simulink model "LCK_DanishV01"  (R2018b)
settings: Solver=FixedStepDiscrete  StartTime=0.0  StopTime=inf  FixedStep=0.01  RelTol=1e-3
PostLoadFcn:
  | if any(exist('dsrtsu_mdlpostloadfcn', 'file') ~= 0), dsrtsu_mdlpostloadfcn('Execute', bdroot); end
values from neighbouring files (symbols this model uses):
  C_DEG2RAD = 0.0175    [LCK_Macro.sldd]
  C_KPH2MPS = 0.2778    [LCK_Macro.sldd]
  C_NEARZERO = 0.0001    [LCK_Macro.sldd]
  C_ONE = 1.0    [LCK_Macro.sldd]
  C_RAD2DEG = 57.2958    [LCK_Macro.sldd]
  C_ZERO = 0.0    [LCK_Macro.sldd]
  k_accel_pedal_pos_per_speed_x : value not decoded    [LCK_LogicPara.sldd]
  k_accel_pedal_pos_per_speed_z : value not decoded    [LCK_LogicPara.sldd]
  k_brake_suprress_hold = 1000.0    [LCK_LogicPara.sldd]
  k_driver_appl_torque_filt = 50.0    [LCK_LogicPara.sldd]
  k_driver_suppression_hold_time = 3000.0    [LCK_LogicPara.sldd]
  k_hands_on_wheel_hold_msec = 500.0    [LCK_LogicPara.sldd]
  k_hands_on_wheel_torque_hi = 0.2    [LCK_LogicPara.sldd]
  k_hands_on_wheel_torque_lo = 0.15    [LCK_LogicPara.sldd]
  k_handsoff_delay_cycles = 50.0    [LCK_LogicPara.sldd]
  k_handsoff_torq_Lo_CR = 0.3    [LCK_LogicPara.sldd]
  k_handson_delay_cycles = 5.0    [LCK_LogicPara.sldd]
  k_HighAccel_suppress_hold = 3000.0    [LCK_LogicPara.sldd]
  k_HLR_suprress_hold = 3000.0    [LCK_LogicPara.sldd]
  k_hs_StrAng_CR_threshold_z : value not decoded    [LCK_LogicPara.sldd]
  k_LC_Exit_Switch = 0.0    [LCK_LogicPara.sldd]
  k_LCG_Configured = 1.0    [LCK_LogicPara.sldd]
  k_LCK_A0_Rdy2Act_UseConst = 0.0    [LCK_LogicPara.sldd]
  k_LCK_A0Fac_ActSta : value not decoded    [LCK_CtrlPara.sldd]
  k_LCK_A0Fac_DrvStm : value not decoded    [LCK_CtrlPara.sldd]
  k_LCK_A0Shift_LftCurv : value not decoded    [LCK_CtrlPara.sldd]
  k_LCK_A0Shift_RgtCurv : value not decoded    [LCK_CtrlPara.sldd]
  k_LCK_A0Shift_StraLan = 0.0    [LCK_CtrlPara.sldd]
  k_LCK_A0ShiftFac_Dy_LftCurv : value not decoded    [LCK_CtrlPara.sldd]
  k_LCK_A0ShiftFac_Dy_RgtCurv : value not decoded    [LCK_CtrlPara.sldd]
  k_LCK_A0ShiftFac_Vspd : value not decoded    [LCK_CtrlPara.sldd]
  k_LCK_accel_inhibit_thold = 35.0    [LCK_LogicPara.sldd]
  k_LCK_Active2Ready_Mask = 255.0    [LCK_LogicPara.sldd]
  k_LCK_CvatRateBks : value not decoded    [LCK_CtrlPara.sldd]
  k_LCK_CvatrBks : value not decoded    [LCK_CtrlPara.sldd]
  k_LCK_DFac_Dy : value not decoded    [LCK_CtrlPara.sldd]
  k_LCK_DFac_Dy_Curv : value not decoded    [LCK_CtrlPara.sldd]
  k_LCK_DFac_HaCurCen : value not decoded    [LCK_CtrlPara.sldd]
  k_LCK_DFac_HaCurSid : value not decoded    [LCK_CtrlPara.sldd]
  k_LCK_DFac_HadCurCen : value not decoded    [LCK_CtrlPara.sldd]
  k_LCK_DFac_HadCurSid : value not decoded    [LCK_CtrlPara.sldd]
  k_LCK_DFac_HadStrCen : value not decoded    [LCK_CtrlPara.sldd]
  k_LCK_DFac_HadStrSid : value not decoded    [LCK_CtrlPara.sldd]
  k_LCK_DFac_HaStrCen : value not decoded    [LCK_CtrlPara.sldd]
  k_LCK_DFac_HaStrSid : value not decoded    [LCK_CtrlPara.sldd]
  k_LCK_DFac_Rad : value not decoded    [LCK_CtrlPara.sldd]
  k_LCK_DFac_SA_CurCen : value not decoded    [LCK_CtrlPara.sldd]
  k_LCK_DFac_SA_CurSid : value not decoded    [LCK_CtrlPara.sldd]
  k_LCK_DFac_SA_StrCen : value not decoded    [LCK_CtrlPara.sldd]
  k_LCK_DFac_SA_StrSid : value not decoded    [LCK_CtrlPara.sldd]
  k_LCK_DFac_SS_CurCen : value not decoded    [LCK_CtrlPara.sldd]
  k_LCK_DFac_SS_CurSid : value not decoded    [LCK_CtrlPara.sldd]
  k_LCK_DFac_SS_StrCen : value not decoded    [LCK_CtrlPara.sldd]
  k_LCK_DFac_SS_StrSid : value not decoded    [LCK_CtrlPara.sldd]
  k_LCK_DFac_Vspd : value not decoded    [LCK_CtrlPara.sldd]
  k_LCK_DlyTm_DrvStim = 0.2    [LCK_CtrlPara.sldd]
  k_LCK_DTermMax = 2.0    [LCK_CtrlPara.sldd]
  k_LCK_DyBks_Curv : value not decoded    [LCK_CtrlPara.sldd]
  k_LCK_Enable_POOnly = 1.0    [LCK_LogicPara.sldd]
  k_LCK_Entry_DistBuffer = 0.1    [LCK_LogicPara.sldd]
  k_LCK_Fac_Vspd2RngThr_FalRec = 0.23    [LCK_CtrlPara.sldd]
  k_LCK_Ffw_CvatSwh = 0.0    [LCK_CtrlPara.sldd]
  k_LCK_Ffw_DyBks : value not decoded    [LCK_CtrlPara.sldd]
  k_LCK_Ffw_TimCon_CmdFlt = 0.0    [LCK_CtrlPara.sldd]
  k_LCK_FfwDeltaFac_Rad_Lft : value not decoded    [LCK_CtrlPara.sldd]
  k_LCK_FfwDeltaFac_Rad_Rgt : value not decoded    [LCK_CtrlPara.sldd]
  k_LCK_FfwDeltaFac_Vspd : value not decoded    [LCK_CtrlPara.sldd]
  k_LCK_FfwFac_CvatRate_Lft : value not decoded    [LCK_CtrlPara.sldd]
  k_LCK_FfwFac_CvatRate_Rgt : value not decoded    [LCK_CtrlPara.sldd]
  k_LCK_FfwFac_Dy : value not decoded    [LCK_CtrlPara.sldd]
  k_LCK_FfwFac_Rad_Lft : value not decoded    [LCK_CtrlPara.sldd]
  k_LCK_FfwFac_Rad_Rgt : value not decoded    [LCK_CtrlPara.sldd]
  k_LCK_FfwFac_Vspd : value not decoded    [LCK_CtrlPara.sldd]
  k_LCK_FfwTorq_Cvat : value not decoded    [LCK_CtrlPara.sldd]
  k_LCK_HAFac_ActSta : value not decoded    [LCK_CtrlPara.sldd]
  k_LCK_HAFac_DrvStm : value not decoded    [LCK_CtrlPara.sldd]
  k_LCK_HaloTime = 2000.0    [LCK_LogicPara.sldd]
  k_LCK_HaloTime_Switch = 0.0    [LCK_LogicPara.sldd]
  k_LCK_HARFac_ActSta : value not decoded    [LCK_CtrlPara.sldd]
  k_LCK_HARFac_DrvStm : value not decoded    [LCK_CtrlPara.sldd]
  k_LCK_Hed_DyBks : value not decoded    [LCK_CtrlPara.sldd]
  k_LCK_HedAngDiffX : value not decoded    [LCK_CtrlPara.sldd]
  k_LCK_HedAngRateDiffX : value not decoded    [LCK_CtrlPara.sldd]
  k_LCK_HndsOnWhel_DlyTm_Idl2Rdy = 0.0    [LCK_LogicPara.sldd]
  k_LCK_host_veh_width = 1.86    [LCK_LogicPara.sldd]
  k_LCK_Idle2Ready_Mask = 239.0    [LCK_LogicPara.sldd]
  k_LCK_Junc_SusTime = 1.0    [LCK_LogicPara.sldd]
  k_LCK_KpKdDecSlopeLmt = 10.0    [LCK_CtrlPara.sldd]
  k_LCK_KpKdIncSlopeLmt = 5.0    [LCK_CtrlPara.sldd]
  k_LCK_Lat_Ctrl_DFac_Lft = 1.0    [LCK_CtrlPara.sldd]
  k_LCK_Lat_Ctrl_DFac_Rgt = 1.05    [LCK_CtrlPara.sldd]
  k_LCK_Lat_Ctrl_Kd = 0.8    [LCK_CtrlPara.sldd]
  k_LCK_Lat_Ctrl_Ki = 0.5    [LCK_CtrlPara.sldd]
  k_LCK_Lat_Ctrl_Kp = 0.7    [LCK_CtrlPara.sldd]
  k_LCK_Lat_Ctrl_Kp_NearGain = 0.7    [LCK_CtrlPara.sldd]
  k_LCK_Lat_Ctrl_PFac_Lft = 1.0    [LCK_CtrlPara.sldd]
  k_LCK_Lat_Ctrl_PFac_Rgt = 1.05    [LCK_CtrlPara.sldd]
  k_LCK_Lat_Ctrl_TimCon_CmdFlt = 5.0    [LCK_CtrlPara.sldd]
  k_LCK_Lat_DFac_Rad : value not decoded    [LCK_CtrlPara.sldd]
  k_LCK_Lat_DFac_SS_Cur : value not decoded    [LCK_CtrlPara.sldd]
  k_LCK_Lat_DFac_SS_Str : value not decoded    [LCK_CtrlPara.sldd]
  k_LCK_Lat_DFac_Vspd : value not decoded    [LCK_CtrlPara.sldd]
  k_LCK_Lat_DyBks : value not decoded    [LCK_CtrlPara.sldd]
  k_LCK_Lat_IFac_Rad : value not decoded    [LCK_CtrlPara.sldd]
  k_LCK_Lat_IFac_Vspd : value not decoded    [LCK_CtrlPara.sldd]
  k_LCK_Lat_ILmtFac_Dy_CurvLan : value not decoded    [LCK_CtrlPara.sldd]
  k_LCK_Lat_ILmtFac_Dy_StraLan : value not decoded    [LCK_CtrlPara.sldd]
  k_LCK_Lat_ILmtFac_Rad : value not decoded    [LCK_CtrlPara.sldd]
  k_LCK_Lat_ILmtFac_Rad_NearGain = 1.0    [LCK_CtrlPara.sldd]
  k_LCK_Lat_ILmtFac_Vspd_CurvLan : value not decoded    [LCK_CtrlPara.sldd]
  k_LCK_Lat_ILmtFac_Vspd_StraLan : value not decoded    [LCK_CtrlPara.sldd]
  k_LCK_Lat_ITermLmt_Dy = 1.0    [LCK_CtrlPara.sldd]
  k_LCK_Lat_KpKdDecSlopeLmt = 10.0    [LCK_CtrlPara.sldd]
  k_LCK_Lat_KpKdIncSlopeLmt = 10.0    [LCK_CtrlPara.sldd]
  k_LCK_Lat_PFac_Dy_InnLftCur : value not decoded    [LCK_CtrlPara.sldd]
  k_LCK_Lat_PFac_Dy_InnRgtCur : value not decoded    [LCK_CtrlPara.sldd]
  k_LCK_Lat_PFac_Dy_OutLftCur : value not decoded    [LCK_CtrlPara.sldd]
  k_LCK_Lat_PFac_Dy_OutRgtCur : value not decoded    [LCK_CtrlPara.sldd]
  k_LCK_Lat_PFac_Dy_Str : value not decoded    [LCK_CtrlPara.sldd]
  k_LCK_Lat_PFac_Rad : value not decoded    [LCK_CtrlPara.sldd]
  ... (+153 more)
undefined symbols (not defined in the file or in its folder): k_LCK_CurvBks, K_LCK_SPA0A1A2_LMRngCmp_y
libraries: LateralControl_fcns_lib x58, simulink x24
(part 12 of 47)

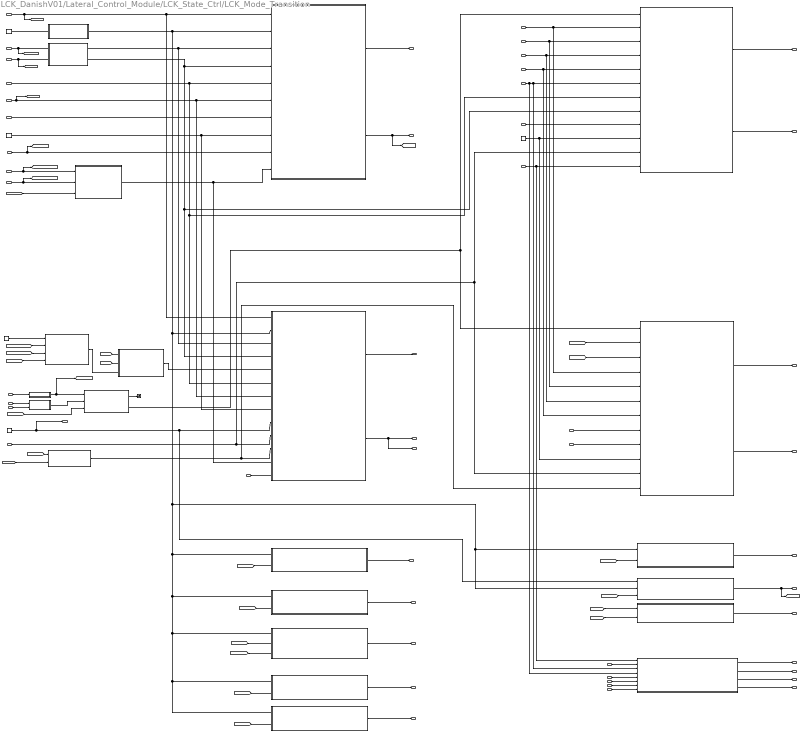
== system LCK_DanishV01/Lateral_Control_Module/LCK_State_Ctrl/LCK_Mode_Transition ==
  Veh_Speed_kph : Inport  Description=_GWMAB30P4.LCK.000_82_
  LDWLKASwReq : Inport  Description=_GWMAB30P4.LCK.000_80_  Port=2
  SP_conf : Inport  Description=_GWMAB30P4.LCK.000_88_  Port=3
  SP_type : Inport  Description=_GWMAB30P4.LCK.000_87_  Port=4
  SPP_A0 : Inport  Description=_GWMAB30P4.LCK.000_111_  Port=5
  SPP_A1 : Inport  Description=_GWMAB30P4.LCK.000_111_  Port=6
  SPP_A2 : Inport  Description=_GWMAB30P4.LCK.000_91_  Port=7
  curr_lane_width : Inport  Description=_GWMAB30P4.LCK.000_90_  Port=8
  VIS_LANE_LEFT_INDIVID_RANGE : Inport  Description=_GACA26P4.LCK.000_5_  Port=9
  VIS_LANE_RIGHT_INDIVID_RANGE : Inport  Description=_GACA26P4.LCK.000_6_  Port=10
  Lin01_Type : Inport  Description=_GWMAB30P4.LCK.000_95_  Port=11
  Lin02_Type : Inport  Port=12
  yaw_deg_iso_filt : Inport  Description=_GWMAB30P4.LCK.000_89_  Port=13
  LKATrqOvrlTrqDStat : Inport  Description=_GWMAB30P4.LCK.000_113_  Port=14
  DirectionIndSwitchPos : Inport  Description=_GWMAB30P4.LCK.000_103_  Port=15
  LCK_Mode : Inport  Description=_GWMAB30P4.LCK.000_112_  Port=16
  LeftLaneChange : Inport  Description=_GWMAB30P4.LCK.000_94_  Port=17
  RightLaneChange : Inport  Description=_GWMAB30P4.LCK.000_95_  Port=18
  f_hands_on_wheel : Inport  Description=_GWMAB30P4.LCK.000_98_  Port=19
  f_driv_override_left : Inport  Description=_GWMAB30P4.LCK.000_96_  Port=20
  f_driv_override_right : Inport  Description=_GWMAB30P4.LCK.000_97_  Port=21
  f_left_driver_suppression : Inport  Description=_GWMAB30P4.LCK.000_110_  Port=22
  f_right_driver_suppression : Inport  Description=_GWMAB30P4.LCK.000_111_  Port=23
  LC_Phase : Inport  Description=_GWMAB30P4.LCK.000_95_  Port=24
  TJA_State : Inport  Description=_GWMAB30P4.LCK.000_80_  Port=25
  ZOP_LCK_Activate : Inport  Description=_GWMAB30P4.LCK.000_80_  Port=26
  ZOP_LC_Command : Inport  Port=27
  PO_Enable : Inport  Port=28
  ACTIVE2READY_Magic_Calculation : Subsystem
  Constant1 : Constant  Tag={'output',{'type','Int32'},'date',737184.60397266201}  Description=_GWMAB30P2.LCK.000_1069_  Value=0
  Constant19 : Constant  Tag={'output',{'type','Int32'},'date',737184.60397266201}  Description=_GWMAB30P2.LCK.000_1069_  Value=0
  Constant3 : Constant  Tag={'output',{'type','Int32'},'date',737184.60397266201}  Description=_GWMAB30P2.LCK.000_1069_  Value=0  OutDataTypeStr=boolean
  Constant4 : Constant  Tag={'output',{'type','Int32'},'date',737184.60397266201}  Description=_GWMAB30P2.LCK.000_1069_
  Constant5 : Constant  Tag={'output',{'type','Int32'},'date',737184.60397266201}  Description=_GWMAB30P2.LCK.000_1069_  Value=0
  Det_LCK_Switch : Subsystem
  Det_TJA_Lat_Req : Subsystem
  Determination_of_ACTIVE2OFF : Subsystem
  Determination_of_ERROR2IDLE : Subsystem
  Determination_of_ERROR2OFF : Subsystem
  Determination_of_ERROR2READY : Subsystem
  Determination_of_IDLE2OFF : Subsystem
  Determination_of_Junction : Subsystem
  Determination_of_Lat_Ctrl_Req : Subsystem
  Determination_of_OFF2IDLE : Subsystem
  Determination_of_OFF2READY : Subsystem
  Determination_of_READY2OFF : Subsystem
  Determination_of_SPP_Valid : Subsystem
  Determination_of_Short_LM_Range : Subsystem
  Determination_of_TJA_Switch : Subsystem
  IDLE2READY_Magic_Calculation : Subsystem
  READY2ACTIVE_Magic_Claculation : Subsystem
  READY2IDLE_Magic_Calculation : Subsystem
  SP_conf_Judgement : Subsystem
  Subsystem : Subsystem
  Terminator : Terminator
  Yaw_Rate_Judgement : Subsystem
  OFF2IDLE : Outport  Description=_GWMAB30P4.LCK.000_187_
  OFF2READY : Outport  Description=_GWMAB30P4.LCK.000_188_  Port=2
  IDLE2OFF : Outport  Description=_GWMAB30P4.LCK.000_190_  Port=3
  IDLE2READY : Outport  Description=_GWMAB30P4.LCK.000_191_  Port=4
  READY2OFF : Outport  Description=_GWMAB30P4.LCK.000_192_  Port=5
  READY2IDLE : Outport  Description=_GWMAB30P4.LCK.000_193_  Port=6
  READY2ACTIVE : Outport  Description=_GWMAB30P4.LCK.000_194_  Port=7
  ACTIVE2OFF : Outport  Description=_GWMAB30P4.LCK.000_192_  Port=8
  ACTIVE2IDLE : Outport  Description=_GWMAB30P4.LCK.000_193_  Port=9
  ACTIVE2READY : Outport  Description=_GWMAB30P4.LCK.000_197_  Port=10
  ERROR2OFF : Outport  Description=_GWMAB30P4.LCK.000_198_  Port=11
  ERROR2IDLE : Outport  Description=_GWMAB30P4.LCK.000_199_  Port=12
  ERROR2READY : Outport  Description=_GWMAB30P4.LCK.000_200_  Port=13
  ERROR_CONDITION : Outport  Description=_GWMAB30P4.LCK.000_193_  Port=14
  LCK2LEFTLC : Outport  Description=_GWMAB30P4.LCK.000_200_  Port=15
  LCK2RIGHTLC : Outport  Description=_GWMAB30P4.LCK.000_200_  Port=16
  LEFTLC2LCK : Outport  Description=_GWMAB30P4.LCK.000_200_  Port=17
  RIGHTLC2LCK : Outport  Description=_GWMAB30P4.LCK.000_200_  Port=18
  IDLE2READY_Magic_Out : Outport  Description=_GWMAB30P4.LCK.000_204_  Port=19
  READY2IDLE_Magic_Out : Outport  Description=_GWMAB30P4.LCK.000_205_  Port=20
  READY2ACTIVE_Magic_Out : Outport  Description=_GWMAB30P4.LCK.000_206_  Port=21
  ACTIVE2READY_Magic_Out : Outport  Description=_GWMAB30P4.LCK.000_207_  Port=22
  wires:
  [SP_type] -> Determination_of_Junction/4(SP_type)
  VIS_LANE_LEFT_INDIVID_RANGE/1 -> [VIS_LANE_LEFT_INDIVID_RANGE], Determination_of_Short_LM_Range/1(VIS_LANE_LEFT_INDIVID_RANGE)
  Determination_of_TJA_Switch/1(TJA_Switch) -> READY2IDLE_Magic_Calculation/2(TJA_Switch), Determination_of_ERROR2IDLE/2(TJA_Switch), Determination_of_ERROR2OFF/1(TJA_Switch), Determination_of_OFF2IDLE/1(TJA_Switch), Determination_of_IDLE2OFF/1(TJA_Switch), Determination_of_OFF2READY/1(TJA_Switch), Determination_of_READY2OFF/1(TJA_Switch), Determination_of_ACTIVE2OFF/1(TJA_Switch), IDLE2READY_Magic_Calculation/2(TJA_Switch)
  Veh_Speed_kph/1 -> [veh_speed_kph], READY2IDLE_Magic_Calculation/1(veh_speed_kph), IDLE2READY_Magic_Calculation/1(Veh_Speed_kph)
  READY2ACTIVE_Magic_Claculation/1(READY2ACTIVE_Magic_Out) -> READY2ACTIVE_Magic_Out/1
  [veh_speed_kph] -> ACTIVE2READY_Magic_Calculation/3(veh_speed_kph)
  IDLE2READY_Magic_Calculation/2(IDLE2READY) -> [IDLE2READY], IDLE2READY/1
  Constant3/1 -> ERROR_CONDITION/1, Determination_of_ERROR2IDLE/1(ERROR_CONDITION), READY2IDLE_Magic_Calculation/9(ERROR_CONDITION)
  Constant5/1 -> ACTIVE2READY_Magic_Calculation/10(ELK_Mode), READY2ACTIVE_Magic_Claculation/10(ELK_Mode)
  TJA_State/1 -> Det_TJA_Lat_Req/1(TJA_State)
  LKATrqOvrlTrqDStat/1 -> READY2IDLE_Magic_Calculation/10(LKATrqOvrlTrqDStat), ACTIVE2READY_Magic_Calculation/11(LKATrqOvrlTrqDStat), READY2ACTIVE_Magic_Claculation/11(LKATrqOvrlTrqDStat)
  Yaw_Rate_Judgement/1(YawRate_Over_Threshold) -> ACTIVE2READY_Magic_Calculation/12(YawRate_Over_Threshold), READY2IDLE_Magic_Calculation/11(YawRate_Over_Threshold)
  f_right_driver_suppression/1 -> ACTIVE2READY_Magic_Calculation/7(f_right_driver_suppression), READY2ACTIVE_Magic_Claculation/5(f_right_driver_suppression)
  yaw_deg_iso_filt/1 -> [yaw_deg_iso_filt], IDLE2READY_Magic_Calculation/9(yaw_deg_iso_filt)
  Determination_of_Short_LM_Range/1(Short_LM_Range) -> READY2IDLE_Magic_Calculation/12(Short_LM_Range), IDLE2READY_Magic_Calculation/10(Short_LM_Range)
  Determination_of_SPP_Valid/1(SP_valid_low_spd) -> READY2IDLE_Magic_Calculation/3(SP_valid_low_spd), IDLE2READY_Magic_Calculation/3(SP_valid_low_spd)
  Determination_of_SPP_Valid/2(SP_valid_high_spd) -> READY2IDLE_Magic_Calculation/4(SP_valid_high_spd), READY2ACTIVE_Magic_Claculation/8(SP_valid_high_spd), IDLE2READY_Magic_Calculation/4(SP_valid_high_spd)
  Determination_of_OFF2READY/1(OFF2READY) -> OFF2READY/1
  Constant4/1 -> READY2IDLE_Magic_Calculation/8(LCK_Feature_Enabled), IDLE2READY_Magic_Calculation/8(LCK_Feature_Enabled)
  curr_lane_width/1 -> READY2IDLE_Magic_Calculation/6(curr_lane_width), READY2ACTIVE_Magic_Claculation/7(curr_lane_width), IDLE2READY_Magic_Calculation/5(curr_lane_width)
  [veh_speed_kph] -> SP_conf_Judgement/1(veh_speed_kph)
  SPP_A2/1 -> [SPP_A2], READY2IDLE_Magic_Calculation/7(SPP_A2), IDLE2READY_Magic_Calculation/6(SPP_A2)
  LCK_Mode/1 -> Subsystem/1(LCK_Mode), READY2ACTIVE_Magic_Claculation/12(LCK_Mode)
  [VIS_LANE_RIGHT_INDIVID_RANGE] -> Determination_of_Junction/3(VIS_LANE_RIGHT_INDIVID_RANGE)
  Constant1/1 -> Determination_of_Junction/1(SP_max_range)
  [yaw_deg_iso_filt] -> Yaw_Rate_Judgement/1(yaw_deg_iso_filt)
  f_hands_on_wheel/1 -> IDLE2READY_Magic_Calculation/7(f_hands_on_wheel)
  RightLaneChange/1 -> ACTIVE2READY_Magic_Calculation/9(RightLaneChange)
  LeftLaneChange/1 -> ACTIVE2READY_Magic_Calculation/8(LeftLaneChange)
  [SPP_A2] -> Yaw_Rate_Judgement/2(SP_A2)
  READY2ACTIVE_Magic_Claculation/2(READY2ACTIVE) -> READY2ACTIVE/1
  [SP_conf] -> SP_conf_Judgement/2(SP_conf)
  Determination_of_ERROR2OFF/1(ERROR2OFF) -> ERROR2OFF/1
  Determination_of_Lat_Ctrl_Req/2(TJA_LatCtrl_Rq) -> ACTIVE2READY_Magic_Calculation/1(TJA_LatCtrl_Rq), READY2ACTIVE_Magic_Claculation/1(TJA_LatCtrl_Rq)
  SP_conf/1 -> [SP_conf], Determination_of_SPP_Valid/2(SP_conf)
  IDLE2READY_Magic_Calculation/1(IDLE2READY_Magic_Out) -> IDLE2READY_Magic_Out/1
  Determination_of_ERROR2IDLE/1(ERROR2IDLE) -> ERROR2IDLE/1, [ERROR2IDLE]
  VIS_LANE_RIGHT_INDIVID_RANGE/1 -> [VIS_LANE_RIGHT_INDIVID_RANGE], Determination_of_Short_LM_Range/2(VIS_LANE_RIGHT_INDIVID_RANGE)
  f_driv_override_left/1 -> ACTIVE2READY_Magic_Calculation/4(f_driv_override_left), READY2ACTIVE_Magic_Claculation/2(f_driv_override_left)
  READY2IDLE_Magic_Calculation/2(READY2IDLE) -> ACTIVE2IDLE/1, READY2IDLE/1
  f_left_driver_suppression/1 -> ACTIVE2READY_Magic_Calculation/6(f_left_driver_suppression), READY2ACTIVE_Magic_Claculation/4(f_left_driver_suppression)
  ACTIVE2READY_Magic_Calculation/1(ACTIVE2READY_Magic_Out) -> ACTIVE2READY_Magic_Out/1
  [veh_speed_kph] -> Determination_of_Lat_Ctrl_Req/3(veh_speed_kph)
  SPP_A0/1 -> Subsystem/4(SPP_A1), Subsystem/3(SPP_A0), READY2ACTIVE_Magic_Claculation/6(SPP_A0)
  [VIS_LANE_LEFT_INDIVID_RANGE] -> Determination_of_Junction/2(VIS_LANE_LEFT_INDIVID_RANGE)
  READY2IDLE_Magic_Calculation/1(READY2IDLE_Magic_Out) -> READY2IDLE_Magic_Out/1
  ACTIVE2READY_Magic_Calculation/2(ACTIVE2READY) -> ACTIVE2READY/1
  f_driv_override_right/1 -> ACTIVE2READY_Magic_Calculation/5(f_driv_override_right), READY2ACTIVE_Magic_Claculation/3(f_driv_override_right)
  Determination_of_READY2OFF/1(READY2OFF) -> READY2OFF/1
  Determination_of_ERROR2READY/1(ERROR2READY) -> ERROR2READY/1
  [veh_speed_kph] -> Determination_of_Short_LM_Range/3(veh_speed_kph)
  Determination_of_IDLE2OFF/1(IDLE2OFF) -> IDLE2OFF/1
  [IDLE2READY] -> Determination_of_OFF2READY/3(IDLE2READY)
  [LCK_Switch] -> ACTIVE2READY_Magic_Calculation/2(LCK_Switch)
  [IDLE2READY] -> Determination_of_ERROR2READY/2(IDLE2READY)
  SP_type/1 -> [SP_type], Determination_of_SPP_Valid/1(SP_type)
  [ERROR2IDLE] -> Determination_of_ERROR2READY/1(ERROR2IDLE)
  SP_conf_Judgement/1(SP_conf_Judgement) -> READY2IDLE_Magic_Calculation/5(SP_conf_Judgement)
  Determination_of_OFF2IDLE/1(OFF2IDLE) -> OFF2IDLE/1
  Constant19/1 -> Determination_of_TJA_Switch/1(TJA_Switch_Input)
  SPP_A1/1 -> READY2ACTIVE_Magic_Claculation/9(SPP_A1)
  Determination_of_Junction/1(Junction) -> SP_conf_Judgement/3(Junction)
  Determination_of_ACTIVE2OFF/1(ACTIVE2OFF) -> ACTIVE2OFF/1
  Determination_of_Lat_Ctrl_Req/1(LCKON_TJAOFF) -> Terminator/1
  Det_LCK_Switch/1(LCK_Switch) -> [LCK_Switch], Determination_of_Lat_Ctrl_Req/1(LCK_Switch)
  LDWLKASwReq/1 -> Det_LCK_Switch/1(LDWLKASwReq)
  [LCK_Switch] -> Determination_of_OFF2IDLE/2(LCK_Switch)
  [LCK_Switch] -> Determination_of_IDLE2OFF/2(LCK_Switch)
  [LCK_Switch] -> Determination_of_OFF2READY/2(LCK_Switch)
  [LCK_Switch] -> Determination_of_READY2OFF/2(LCK_Switch)
  [LCK_Switch] -> Determination_of_ACTIVE2OFF/2(LCK_Switch)
  [LCK_Switch] -> Determination_of_ERROR2OFF/2(LCK_Switch)
  [LCK_Switch] -> Determination_of_ERROR2IDLE/3(LCK_Switch)
  DirectionIndSwitchPos/1 -> Subsystem/2(DirectionIndSwitchPos)
  LC_Phase/1 -> Subsystem/5(LC_Phase)
  Subsystem/1(LCK2LEFTLC) -> LCK2LEFTLC/1
  Subsystem/2(LCK2RIGHTLC) -> LCK2RIGHTLC/1
  Subsystem/3(LEFTLC2LCK) -> LEFTLC2LCK/1
  Subsystem/4(RIGHTLC2LCK) -> RIGHTLC2LCK/1
  Det_TJA_Lat_Req/1(TJA_Lat_Req) -> Determination_of_Lat_Ctrl_Req/2(TJA_LatCtrl_Rq_Input)
  ZOP_LCK_Activate/1 -> Det_TJA_Lat_Req/2(ZOP_LCK_Activate)
  ZOP_LC_Command/1 -> Subsystem/6(ZOP_LC_Command)
  Lin01_Type/1 -> Subsystem/7(Lin01_Type)
  Lin02_Type/1 -> Subsystem/8(Lin02_Type)
  PO_Enable/1 -> READY2IDLE_Magic_Calculation/13(PO_Enable)
